simulink model "Simulation_Fahrmodell_v3_straight_line"  (R2023b)
settings: Solver=ode14x  StartTime=0.0  StopTime=600  FixedStep=0.005  RelTol=1e-3
values from neighbouring files (symbols this model uses):
  bat = bat.computePack()    [DoE_main_sensitivity.m]
  cp = cp.computeP4Map(P4, E2, P4_DM, E3, E4)    [DoE_main_sensitivity.m]
  gb = gb.computeShiftMaps()    [DoE_main_sensitivity.m]
  Ice_derfacLoadDecrease_MAP = Ice_derfacLoadDecrease_base    [setup_turbo.m]
  Ice_derfacLoadIncrease_MAP = Ice_derfacLoadIncrease_base    [setup_turbo.m]
  Ice_n_axis = [500, 1000, 1100, 1250, 1320, 1500, 1750, 2000, 2500, 3000, 4500, 6000]    [setup_turbo.m]
  Ice_relLoadMax_CUR_n = [500, 6000]    [setup_turbo.m]
  Ice_relLoadMax_CUR_val = [1.0,  1.0]    [setup_turbo.m]
  Ice_rl_axis_norm = [0.0000, 0.4430, 0.5700, 0.6330, 0.6960, 0.7590, 0.8230, 0.8860, 0.9490, 1.0000]    [setup_turbo.m]
  P4 = cfgNum(cfg, 'P4', 0)    [DoE_main_sensitivity.m]
  P4_DM = cfgNum(cfg, 'P4_DM', 0)    [DoE_main_sensitivity.m]
  pt = pt.setupHybrid()    [DoE_main_sensitivity.m]
  slip_pacejka =     [init_slip.mat]
  use_turbo_model = 0    [setup_turbo.m]
  veh = VehicleConfig()    [DoE_main_sensitivity.m]
undefined symbols (not defined in the file or in its folder): cp_Zelle_JpkgK, seconds, SKO_STREET_CHAL, SKO_WHEEL_TYP_CHAL, T_init_degC, Track, TT_sliced, v_Fzg_init_kmph
libraries: nesl_utility x15, fl_lib x9, simulink x4
(part 4 of 6)

== system Simulation_Fahrmodell_v3_straight_line/Vehicle Dynamics Model /Drivetrain/Primary and Secondary Axle Powertrain Selector/Secondary Axle Powertrain Selector/Auswahl P4, P4_Dual-Motor/No Secondary Axle ==
  n_mot_Upmin : Inport
  Regelfaktor1 : Inport  Port=2
  iAG : Inport  Port=3
  i_ges : Inport  Port=4
  Torque_sh : Inport  Port=5
  Constant : Constant  Value=0
  Terminator{,1..4} (5 alike) : Terminator
  M_Nm GET P4 : Outport
  wires:
  Constant/1 -> M_Nm GET P4/1
  i_ges/1 -> Terminator/1
  iAG/1 -> Terminator1/1
  Regelfaktor1/1 -> Terminator2/1
  n_mot_Upmin/1 -> Terminator3/1
  Torque_sh/1 -> Terminator4/1

== system Simulation_Fahrmodell_v3_straight_line/Vehicle Dynamics Model /Drivetrain/Primary and Secondary Axle Powertrain Selector/Secondary Axle Powertrain Selector/Auswahl P4, P4_Dual-Motor/P4 // E2 Single Motor ==
  n_mot_Upmin : Inport
  Regelfaktor1 : Inport  Port=2
  iAG : Inport  Port=3
  i_ges : Inport  Port=4
  Torque_sh : Inport  Port=5
  1-D Lookup Table1 : Lookup_n-D  NumberOfTableDimensions=1  BreakpointsForDimension1=cp.speed_breakpoints_P4  Table=cp.torque_values_P4  InternalRulePriority=Speed  RndMeth=Simplest
  AG Übersetzung : Product
  Battery and Operating Strategy Limitation (Drive) : Subsystem
  Battery and Operating Strategy Limitation (Recuperation) : Subsystem
  Bus Selector : BusSelector  OutputSignals=tq_sh_P4_des
  Constant : Constant  Value=gb.i_ges_P4
  Constant1 : Constant  Value=gb.i_ges_P4
  Constant5 : Constant  Value=0
  Divide : Product  Inputs=*/
  Gain : Gain  Gain=-1
  Min : MinMax  Inputs=2
  Power Calculation : Subsystem
  "Power Calculation " : Subsystem
  Product : Product
  Relational Operator1 : RelationalOperator  OutDataTypeStr=boolean  RndMeth=Simplest  InputSameDT=off
  Saturation : Saturate  UpperLimit=inf  LowerLimit=0
  Saturation1 : Saturate  UpperLimit=inf  LowerLimit=1
  Smoothing Logic sanfterer Übergang1 : TransferFcn  Denominator=[0.17 1]
  Switch1 : Switch  Criteria=u2 > Threshold  SaturateOnIntegerOverflow=off  InputSameDT=off
  Terminator : Terminator
  M_Nm GET P4 : Outport
  tag scope: P_max_EM_P4_kW=global, P_min_EM_P4_kW=global, tq_sh_P4_max=global
  wires:
  Regelfaktor1/1 -> Relational Operator1/1  "Regelfaktor1"
  Smoothing Logic sanfterer Übergang1/1 -> AG Übersetzung/2
  Relational Operator1/1 -> Switch1/2
  Constant5/1 -> Relational Operator1/2
  Switch1/1 -> Smoothing Logic sanfterer Übergang1/1  "Gesamtmoment motorseitig"
  AG Übersetzung/1 -> M_Nm GET P4/1
  Constant/1 -> AG Übersetzung/1
  iAG/1 -> Terminator/1  "iAG"
  i_ges/1 -> Saturation1/1
  Power Calculation/1(P_kW) -> [P_max_EM_P4_kW]  "P_max_EM_P4_kW"
  Bus Selector/1 -> Saturation/1  "<tq_sh_P4_des>"
  Product/1 -> Battery and Operating Strategy Limitation (Recuperation)/1(Motordrehzahl (1/min)), Battery and Operating Strategy Limitation (Drive)/1(Motordrehzahl (1/min)), 1-D Lookup Table1/1  "Motordrehzahl (1/min)"
  Saturation/1 -> Min/2
  "Power Calculation "/1(P_kW) -> [P_min_EM_P4_kW]  "P_min_EM_P4_kW"
  1-D Lookup Table1/1 -> Gain/1, [tq_sh_P4_max], Min/1
  Torque_sh/1 -> Bus Selector/1
  n_mot_Upmin/1 -> Divide/1  "Motordrehzahl (1/min)"
  Divide/1 -> Product/1  "Motordrehzahl (1/min)"
  Constant1/1 -> Product/2
  Saturation1/1 -> Divide/2
  Battery and Operating Strategy Limitation (Drive)/2(tq_sh_P4_bat_limted) -> Switch1/1, Power Calculation/2(tq_sh_P4_bat_limted)
  Min/1 -> Battery and Operating Strategy Limitation (Drive)/2(Torque_Drive_In)
  [P_max_EM_kW] -> Battery and Operating Strategy Limitation (Drive)/3(P_max_EV_kW)  "P_max_EM_kW"
  Battery and Operating Strategy Limitation (Drive)/1(n_Upmin OUT) -> Power Calculation/1(n_Upmin)
  Battery and Operating Strategy Limitation (Recuperation)/2(tq_sh_P4_bat_limted_recu) -> Switch1/3, "Power Calculation "/2(tq_sh_P4_bat_limted_recu)
  Gain/1 -> Battery and Operating Strategy Limitation (Recuperation)/2(Torque_Recu_In)
  [P_min_EM_kW] -> Battery and Operating Strategy Limitation (Recuperation)/3(P_min_EV_kW)  "P_min_EM_kW"
  Battery and Operating Strategy Limitation (Recuperation)/1(n_Upmin OUT) -> "Power Calculation "/1(n_Upmin)

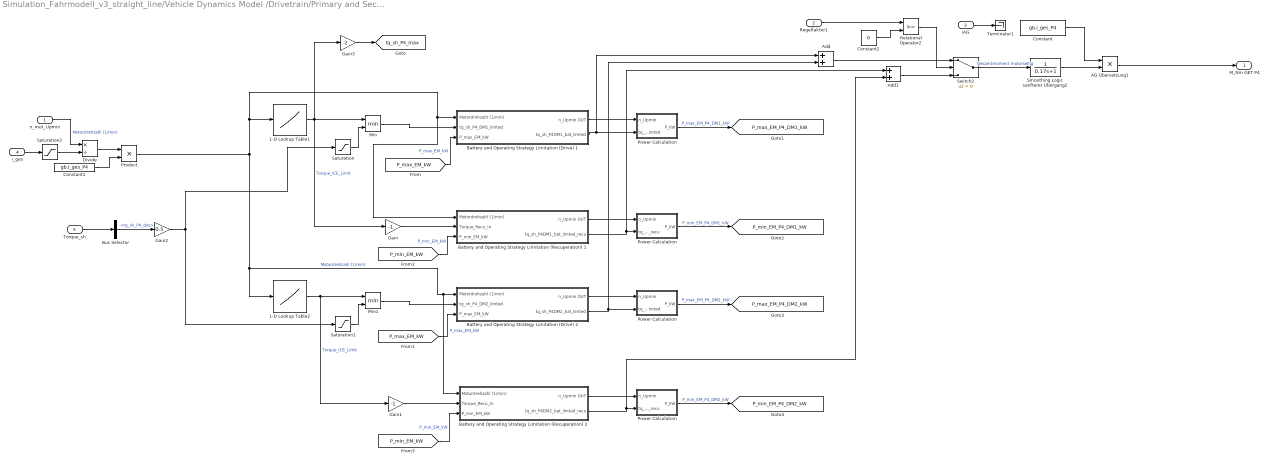
== system Simulation_Fahrmodell_v3_straight_line/Vehicle Dynamics Model /Drivetrain/Primary and Secondary Axle Powertrain Selector/Secondary Axle Powertrain Selector/Auswahl P4, P4_Dual-Motor/P4 // E3 // E4 Dual Motor ==
  n_mot_Upmin : Inport
  Regelfaktor1 : Inport  Port=2
  iAG : Inport  Port=3
  i_ges : Inport  Port=4
  Torque_sh : Inport  Port=5
  1-D Lookup Table1 : Lookup_n-D  NumberOfTableDimensions=1  BreakpointsForDimension1=cp.speed_breakpoints_P4  Table=cp.torque_values_P4  InternalRulePriority=Speed  RndMeth=Simplest
  1-D Lookup Table2 : Lookup_n-D  NumberOfTableDimensions=1  BreakpointsForDimension1=cp.speed_breakpoints_P4  Table=cp.torque_values_P4  InternalRulePriority=Speed  RndMeth=Simplest
  AG Übersetzung1 : Product
  Add : Sum
  Add1 : Sum
  Battery and Operating Strategy Limitation (Drive) 1 : Subsystem
  Battery and Operating Strategy Limitation (Drive) 2 : Subsystem
  Battery and Operating Strategy Limitation (Recuperation) 1 : Subsystem
  Battery and Operating Strategy Limitation (Recuperation) 2 : Subsystem
  Bus Selector : BusSelector  OutputSignals=tq_sh_P4_des
  Constant : Constant  Value=gb.i_ges_P4
  Constant1 : Constant  Value=gb.i_ges_P4
  Constant2 : Constant  Value=0
  Divide : Product  Inputs=*/
  Gain : Gain  Gain=-1
  Gain1 : Gain  Gain=-1
  Gain2 : Gain  Gain=0.5
  Gain3 : Gain  Gain=2
  Min : MinMax  Inputs=2
  Min1 : MinMax  Inputs=2
  "Power Calculation " : Subsystem
  "Power Calculation   " : Subsystem
  "Power Calculation    " : Subsystem
  "Power Calculation     " : Subsystem
  Product : Product
  Relational Operator2 : RelationalOperator  OutDataTypeStr=boolean  RndMeth=Simplest  InputSameDT=off
  Saturation : Saturate  UpperLimit=inf  LowerLimit=0
  Saturation1 : Saturate  UpperLimit=inf  LowerLimit=0
  Saturation2 : Saturate  UpperLimit=inf  LowerLimit=1
  Smoothing Logic sanfterer Übergang2 : TransferFcn  Denominator=[0.17 1]
  Switch2 : Switch  Criteria=u2 > Threshold  SaturateOnIntegerOverflow=off  InputSameDT=off
  Terminator1 : Terminator
  M_Nm GET P4 : Outport
  tag scope: P_max_EM_P4_DM1_kW=global, P_max_EM_P4_DM2_kW=global, P_min_EM_P4_DM1_kW=global, P_min_EM_P4_DM2_kW=global, tq_sh_P4_max=global
  wires:
  Bus Selector/1 -> Gain2/1  "<tq_sh_P4_des>"
  "Power Calculation    "/1(P_kW) -> [P_min_EM_P4_DM1_kW]  "P_min_EM_P4_DM1_kW"
  Torque_sh/1 -> Bus Selector/1
  "Power Calculation     "/1(P_kW) -> [P_max_EM_P4_DM1_kW]  "P_max_EM_P4_DM1_kW"
  1-D Lookup Table1/1 -> Gain3/1, Min/1, Gain/1  "Torque_ICE_Limit"
  Saturation/1 -> Min/2
  "Power Calculation "/1(P_kW) -> [P_min_EM_P4_DM2_kW]  "P_min_EM_P4_DM2_kW"
  "Power Calculation   "/1(P_kW) -> [P_max_EM_P4_DM2_kW]  "P_max_EM_P4_DM2_kW"
  1-D Lookup Table2/1 -> Gain1/1, Min1/1  "Torque_ICE_Limit"
  Saturation1/1 -> Min1/2
  AG Übersetzung1/1 -> M_Nm GET P4/1
  Constant/1 -> AG Übersetzung1/1
  Switch2/1 -> Smoothing Logic sanfterer Übergang2/1  "Gesamtmoment motorseitig"
  iAG/1 -> Terminator1/1
  Relational Operator2/1 -> Switch2/2
  Regelfaktor1/1 -> Relational Operator2/1
  Add1/1 -> Switch2/3
  Constant2/1 -> Relational Operator2/2
  Add/1 -> Switch2/1
  Smoothing Logic sanfterer Übergang2/1 -> AG Übersetzung1/2
  Gain2/1 -> Saturation/1, Saturation1/1
  n_mot_Upmin/1 -> Divide/1  "Motordrehzahl (1/min)"
  i_ges/1 -> Saturation2/1
  Divide/1 -> Product/1
  Constant1/1 -> Product/2
  Product/1 -> Battery and Operating Strategy Limitation (Recuperation) 1/1(Motordrehzahl (1/min)), Battery and Operating Strategy Limitation (Drive) 1/1(Motordrehzahl (1/min)), 1-D Lookup Table1/1, 1-D Lookup Table2/1, Battery and Operating Strategy Limitation (Recuperation) 2/1(Motordrehzahl (1/min)), Battery and Operating Strategy Limitation (Drive) 2/1(Motordrehzahl (1/min))  "Motordrehzahl (1/min)"
  Saturation2/1 -> Divide/2
  Gain3/1 -> [tq_sh_P4_max]
  Battery and Operating Strategy Limitation (Drive) 1/2(tq_sh_P4DM1_bat_limted) -> Add/1, "Power Calculation     "/2(tq_sh_P4DM1_bat_limted)
  Min/1 -> Battery and Operating Strategy Limitation (Drive) 1/2(tq_sh_P4_DM1_limted)
  [P_max_EM_kW] -> Battery and Operating Strategy Limitation (Drive) 1/3(P_max_EM_kW)  "P_max_EM_kW"
  Battery and Operating Strategy Limitation (Drive) 1/1(n_Upmin OUT) -> "Power Calculation     "/1(n_Upmin)
  Battery and Operating Strategy Limitation (Recuperation) 1/2(tq_sh_P4DM1_bat_limted_recu) -> Add1/1, "Power Calculation    "/2(tq_sh_P4DM1_bat_limted_recu)
  Gain/1 -> Battery and Operating Strategy Limitation (Recuperation) 1/2(Torque_Recu_In)
  [P_min_EM_kW] -> Battery and Operating Strategy Limitation (Recuperation) 1/3(P_min_EM_kW)  "P_min_EM_kW"
  Battery and Operating Strategy Limitation (Recuperation) 1/1(n_Upmin OUT) -> "Power Calculation    "/1(n_Upmin)
  Battery and Operating Strategy Limitation (Drive) 2/2(tq_sh_P4DM2_bat_limted) -> Add/2, "Power Calculation   "/2(tq_sh_P4DM2_bat_limted)
  Min1/1 -> Battery and Operating Strategy Limitation (Drive) 2/2(tq_sh_P4_DM2_limted)
  [P_max_EM_kW] -> Battery and Operating Strategy Limitation (Drive) 2/3(P_max_EM_kW)  "P_max_EM_kW"
  Battery and Operating Strategy Limitation (Drive) 2/1(n_Upmin OUT) -> "Power Calculation   "/1(n_Upmin)
  Battery and Operating Strategy Limitation (Recuperation) 2/2(tq_sh_P4DM2_bat_limted_recu) -> Add1/2, "Power Calculation "/2(tq_sh_P4DM2_bat_limted_recu)
  Gain1/1 -> Battery and Operating Strategy Limitation (Recuperation) 2/2(Torque_Recu_In)
  [P_min_EM_kW] -> Battery and Operating Strategy Limitation (Recuperation) 2/3(P_min_EM_kW)  "P_min_EM_kW"
  Battery and Operating Strategy Limitation (Recuperation) 2/1(n_Upmin OUT) -> "Power Calculation "/1(n_Upmin)

== system Simulation_Fahrmodell_v3_straight_line/Vehicle Dynamics Model /Drivetrain/GETRIEBE auswahl VK, EV/Transmission Selector/ICE Multi-Speed/Simulation Doppelkupplung (Gangwechsel ohne Zugkraftunterbrechung) orig2/Vorheriger Wert ==
  In1 : Inport
  Delay : Delay  DelayLength=1
  Memory : Memory
  Relational Operator : RelationalOperator  Operator=~=  OutDataTypeStr=boolean  RndMeth=Simplest  InputSameDT=off
  Switch1 : Switch  Criteria=u2 > Threshold  SaturateOnIntegerOverflow=off  InputSameDT=off
  Out1 : Outport
  wires:
  Switch1/1 -> Memory/1, Out1/1
  Relational Operator/1 -> Switch1/2
  Delay/1 -> Relational Operator/2, Switch1/1
  In1/1 -> Relational Operator/1, Delay/1
  Memory/1 -> Switch1/3

== system Simulation_Fahrmodell_v3_straight_line/Vehicle Dynamics Model /Drivetrain/GETRIEBE auswahl VK, EV/Transmission Selector/ICE Multi-Speed/Subsystem1/Desired Gear  ==
  Current Gear : Inport
  Upshift_Signal : Inport  Port=2
  cmd : Inport  Port=3
  Downshift_Signal : Inport  Port=4
  Add : Sum
  Add1 : Sum  Inputs=+-
  Begrenzung Gang : Saturate  UpperLimit=gb.No_Gears  LowerLimit=1
  Constant1 : Constant
  Constant2 : Constant
  Constant6 : Constant  Value=0
  Relational Operator1 : RelationalOperator  Operator===  OutDataTypeStr=boolean  RndMeth=Simplest  InputSameDT=off
  Switch{1,3..5} (4 alike) : Switch  Criteria=u2 > Threshold  SaturateOnIntegerOverflow=off  InputSameDT=off
  Unit Delay : UnitDelay  SampleTime=0.005
  desiredGear : Outport
  wires:
  Add1/1 -> Switch4/1
  Current Gear/1 -> Add1/1, Switch4/3, Switch3/3, Add/1, Switch1/1
  Switch1/1 -> Begrenzung Gang/1  "Current_Gear"
  Constant1/1 -> Add/2
  Add/1 -> Switch3/1
  Upshift_Signal/1 -> Switch3/2
  Switch4/1 -> Switch5/3
  cmd/1 -> Switch5/2, Relational Operator1/1
  Switch3/1 -> Switch5/1
  Relational Operator1/1 -> Switch1/2
  Unit Delay/1 -> desiredGear/1
  Switch5/1 -> Switch1/3  "Current_Gear"
  Constant6/1 -> Relational Operator1/2
  Constant2/1 -> Add1/2
  Begrenzung Gang/1 -> Unit Delay/1  "Normal"
  Downshift_Signal/1 -> Switch4/2

== system Simulation_Fahrmodell_v3_straight_line/Vehicle Dynamics Model /Drivetrain/GETRIEBE auswahl VK, EV/Transmission Selector/ICE Multi-Speed/Subsystem1/Locktime Bypass Conditions  ==
  note: FOR DOWNSHIFT
  note: FOR UPSHIFT
  Gear upshift Rpm : Inport
  Current Rpm : Inport  Port=2
  Gear downshift Rpm : Inport  Port=3
  AND : Logic  IconShape=distinctive  AllPortsSameDT=off  OutDataTypeStr=boolean
  AND1 : Logic  IconShape=distinctive  AllPortsSameDT=off  OutDataTypeStr=boolean
  AND2 : Logic  IconShape=distinctive  AllPortsSameDT=off  OutDataTypeStr=boolean
  Constant{4..5,7..8} (4 alike) : Constant  Value=0
  OR : Logic  Operator=OR  IconShape=distinctive  AllPortsSameDT=off  OutDataTypeStr=boolean
  OR1 : Logic  Operator=OR  IconShape=distinctive  AllPortsSameDT=off  OutDataTypeStr=boolean
  Relational Operator2 : RelationalOperator  Operator=>  OutDataTypeStr=boolean  RndMeth=Simplest  InputSameDT=off
  Relational Operator5 : RelationalOperator  Operator=<=  OutDataTypeStr=boolean  RndMeth=Simplest  InputSameDT=off
  Relational Operator6 : RelationalOperator  Operator=<=  OutDataTypeStr=boolean  RndMeth=Simplest  InputSameDT=off
  Relational Operator7 : RelationalOperator  OutDataTypeStr=boolean  RndMeth=Simplest  InputSameDT=off
  Relational Operator8 : RelationalOperator  Operator=>  OutDataTypeStr=boolean  RndMeth=Simplest  InputSameDT=off
  Relational Operator9 : RelationalOperator  Operator=<=  OutDataTypeStr=boolean  RndMeth=Simplest  InputSameDT=off
  cmd_Bypass_Lock_time : Outport
  wires:
  Constant8/1 -> Relational Operator9/2
  Relational Operator5/1 -> AND1/1
  [Gaspedalposition] -> Relational Operator5/1, Relational Operator8/1, Relational Operator2/1  "Gas Pedal Position"
  Relational Operator7/1 -> AND/2
  Relational Operator2/1 -> AND/1
  Relational Operator6/1 -> AND1/2
  Gear downshift Rpm/1 -> Relational Operator6/2
  Constant4/1 -> Relational Operator2/2
  Current Rpm/1 -> Relational Operator7/1, Relational Operator6/1
  AND1/1 -> OR/1
  Constant7/1 -> Relational Operator8/2
  OR/1 -> OR1/2  "Bypass Lock time"
  AND/1 -> OR1/1  "Bypass Lock time"
  Constant5/1 -> Relational Operator5/2
  AND2/1 -> OR/2
  Relational Operator8/1 -> AND2/1
  Relational Operator9/1 -> AND2/2
  [S_BUS_IST_Profil_a] -> Relational Operator9/1  "Acceleration"
  OR1/1 -> cmd_Bypass_Lock_time/1  "cmd_Bypass_Lock_time"
  Gear upshift Rpm/1 -> Relational Operator7/2

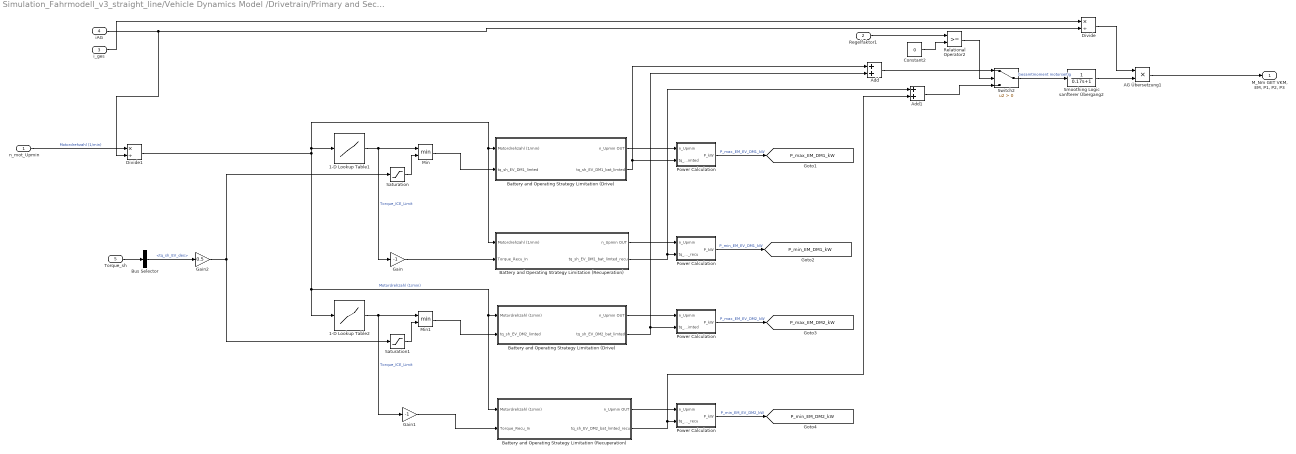
== system Simulation_Fahrmodell_v3_straight_line/Vehicle Dynamics Model /Drivetrain/Primary and Secondary Axle Powertrain Selector/Primary Axle Powertrain Selector/Electric Drive/Variant Subsystem/EV Dual Motor ==
  n_mot_Upmin : Inport
  Regelfaktor1 : Inport  Port=2
  i_ges : Inport  Port=3
  iAG : Inport  Port=4
  Torque_sh : Inport  Port=5
  1-D Lookup Table1 : Lookup_n-D  NumberOfTableDimensions=1  BreakpointsForDimension1=cp.speed_breakpoints_EV  Table=cp.torque_values_EV  InternalRulePriority=Speed  RndMeth=Simplest
  1-D Lookup Table2 : Lookup_n-D  NumberOfTableDimensions=1  BreakpointsForDimension1=cp.speed_breakpoints_EV  Table=cp.torque_values_EV  InternalRulePriority=Speed  RndMeth=Simplest
  AG Übersetzung1 : Product
  Add : Sum
  Add1 : Sum
  Battery and Operating Strategy Limitation (Drive) : Subsystem
  "Battery and Operating Strategy Limitation (Drive) " : Subsystem
  Battery and Operating Strategy Limitation (Recuperation) : Subsystem
  "Battery and Operating Strategy Limitation (Recuperation) " : Subsystem
  Bus Selector : BusSelector  OutputSignals=tq_sh_EV_des
  Constant2 : Constant  Value=0
  Divide : Product  Inputs=*/
  Divide1 : Product  Inputs=*/
  Gain : Gain  Gain=-1
  Gain1 : Gain  Gain=-1
  Gain2 : Gain  Gain=0.5
  Min : MinMax  Inputs=2
  Min1 : MinMax  Inputs=2
  Power Calculation : Subsystem
  "Power Calculation " : Subsystem
  "Power Calculation  " : Subsystem
  "Power Calculation    " : Subsystem
  Relational Operator2 : RelationalOperator  OutDataTypeStr=boolean  RndMeth=Simplest  InputSameDT=off
  Saturation : Saturate  UpperLimit=inf  LowerLimit=0
  Saturation1 : Saturate  UpperLimit=inf  LowerLimit=0
  Smoothing Logic sanfterer Übergang2 : TransferFcn  Denominator=[0.17 1]
  Switch2 : Switch  Criteria=u2 > Threshold  SaturateOnIntegerOverflow=off  InputSameDT=off
  "M_Nm GET VKM, EM, P1, P2, P3" : Outport
  tag scope: P_max_EM_DM1_kW=global, P_max_EM_DM2_kW=global, P_min_EM_DM1_kW=global, P_min_EM_DM2_kW=global
  wires:
  Add1/1 -> Switch2/3
  Add/1 -> Switch2/1
  Switch2/1 -> Smoothing Logic sanfterer Übergang2/1  "Gesamtmoment motorseitig"
  Smoothing Logic sanfterer Übergang2/1 -> AG Übersetzung1/2
  Regelfaktor1/1 -> Relational Operator2/1
  Relational Operator2/1 -> Switch2/2
  AG Übersetzung1/1 -> "M_Nm GET VKM, EM, P1, P2, P3"/1
  Constant2/1 -> Relational Operator2/2
  i_ges/1 -> Divide/1
  iAG/1 -> Divide1/2, Divide/2
  Divide/1 -> AG Übersetzung1/1
  Saturation1/1 -> Min1/2
  "Power Calculation    "/1(P_kW) -> [P_max_EM_DM2_kW]  "P_max_EM_EV_DM2_kW"
  1-D Lookup Table2/1 -> Gain1/1, Min1/1  "Torque_ICE_Limit"
  "Power Calculation  "/1(P_kW) -> [P_min_EM_DM1_kW]  "P_min_EM_EV_DM1_kW"
  "Power Calculation "/1(P_kW) -> [P_max_EM_DM1_kW]  "P_max_EM_EV_DM1_kW"
  Divide1/1 -> 1-D Lookup Table2/1, "Battery and Operating Strategy Limitation (Recuperation) "/1(Motordrehzahl (1/min)), "Battery and Operating Strategy Limitation (Drive) "/1(Motordrehzahl (1/min)), Battery and Operating Strategy Limitation (Recuperation)/1(Motordrehzahl (1/min)), Battery and Operating Strategy Limitation (Drive)/1(Motordrehzahl (1/min)), 1-D Lookup Table1/1  "Motordrehzahl (1/min)"
  Power Calculation/1(P_kW) -> [P_min_EM_DM2_kW]  "P_min_EM_EV_DM2_kW"
  Gain2/1 -> Saturation1/1, Saturation/1
  Saturation/1 -> Min/2
  1-D Lookup Table1/1 -> Gain/1, Min/1  "Torque_ICE_Limit"
  Torque_sh/1 -> Bus Selector/1
  Bus Selector/1 -> Gain2/1  "<tq_sh_EV_des>"
  n_mot_Upmin/1 -> Divide1/1  "Motordrehzahl (1/min)"
  Battery and Operating Strategy Limitation (Drive)/2(tq_sh_EV_DM1_bat_limted) -> Add/1, "Power Calculation "/2(tq_sh_EV_DM1_bat_limted)
  Min/1 -> Battery and Operating Strategy Limitation (Drive)/2(tq_sh_EV_DM1_limted)
  Battery and Operating Strategy Limitation (Drive)/1(n_Upmin OUT) -> "Power Calculation "/1(n_Upmin)
  Battery and Operating Strategy Limitation (Recuperation)/2(tq_sh_EV_DM1_bat_limted_recu) -> Add1/1, "Power Calculation  "/2(tq_sh_EV_DM1_bat_limted_recu)
  Gain/1 -> Battery and Operating Strategy Limitation (Recuperation)/2(Torque_Recu_In)
  Battery and Operating Strategy Limitation (Recuperation)/1(n_Upmin OUT) -> "Power Calculation  "/1(n_Upmin)
  "Battery and Operating Strategy Limitation (Drive) "/2(tq_sh_EV_DM2_bat_limted) -> Add/2, "Power Calculation    "/2(tq_sh_EV_DM2_bat_limted)
  Min1/1 -> "Battery and Operating Strategy Limitation (Drive) "/2(tq_sh_EV_DM2_limted)
  "Battery and Operating Strategy Limitation (Drive) "/1(n_Upmin OUT) -> "Power Calculation    "/1(n_Upmin)
  "Battery and Operating Strategy Limitation (Recuperation) "/2(tq_sh_EV_DM2_bat_limted_recu) -> Add1/2, Power Calculation/2(tq_sh_EV_DM2_bat_limted_recu)
  Gain1/1 -> "Battery and Operating Strategy Limitation (Recuperation) "/2(Torque_Recu_In)
  "Battery and Operating Strategy Limitation (Recuperation) "/1(n_Upmin OUT) -> Power Calculation/1(n_Upmin)

== system Simulation_Fahrmodell_v3_straight_line/Vehicle Dynamics Model /Drivetrain/Primary and Secondary Axle Powertrain Selector/Primary Axle Powertrain Selector/Electric Drive/Variant Subsystem/EV Single Motor ==
  Regelfaktor1 : Inport
  n_mot_Upmin : Inport  Port=2
  i_ges : Inport  Port=3
  iAG : Inport  Port=4
  Torque_sh : Inport  Port=5
  1-D Lookup Table1 : Lookup_n-D  NumberOfTableDimensions=1  BreakpointsForDimension1=cp.speed_breakpoints_EV  Table=cp.torque_values_EV  InternalRulePriority=Speed  RndMeth=Simplest
  Battery and Operating Strategy Limitation (Drive) : Subsystem
  Battery and Operating Strategy Limitation (Recuperation) : Subsystem
  Bus Selector : BusSelector  OutputSignals=tq_sh_EV_des
  Constant7 : Constant  Value=0
  Gain : Gain  Gain=-1
  Min : MinMax  Inputs=2
  Power Calculation : Subsystem
  "Power Calculation " : Subsystem
  Relational Operator2 : RelationalOperator  OutDataTypeStr=boolean  RndMeth=Simplest  InputSameDT=off
  Saturation : Saturate  UpperLimit=inf  LowerLimit=0
  Smoothing Logic sanfterer Übergang2 : TransferFcn  Denominator=[0.17 1]
  Switch2 : Switch  Criteria=u2 > Threshold  SaturateOnIntegerOverflow=off  InputSameDT=off
  Terminator : Terminator
  Wirkungsgrad Antriebsstrang1 : Subsystem
  i_GES Übersetzung : Product
  "M_Nm GET VKM, EM, P1, P2, P3" : Outport
  tag scope: P_max_EM_EV_kW=global, P_min_EM_EV_kW=global
  wires:
  iAG/1 -> Terminator/1
  Constant7/1 -> Relational Operator2/2
  Smoothing Logic sanfterer Übergang2/1 -> i_GES Übersetzung/2
  Switch2/1 -> Smoothing Logic sanfterer Übergang2/1  "Gesamtmoment motorseitig"
  Wirkungsgrad Antriebsstrang1/1(M_Nm OUT) -> "M_Nm GET VKM, EM, P1, P2, P3"/1
  Relational Operator2/1 -> Switch2/2
  Regelfaktor1/1 -> Relational Operator2/1
  i_GES Übersetzung/1 -> Wirkungsgrad Antriebsstrang1/1(M_Nm IN)
  i_ges/1 -> i_GES Übersetzung/1  "i_GES"
  n_mot_Upmin/1 -> Battery and Operating Strategy Limitation (Recuperation)/1(Motordrehzahl (1/min)), Battery and Operating Strategy Limitation (Drive)/1(Motordrehzahl (1/min)), 1-D Lookup Table1/1  "Motordrehzahl (1/min)"
  Power Calculation/1(P_kW) -> [P_max_EM_EV_kW]  "P_max_EM_EV_kW"
  1-D Lookup Table1/1 -> Min/1, Gain/1  "Torque_ICE_Limit"
  Saturation/1 -> Min/2
  Bus Selector/1 -> Saturation/1  "<tq_sh_EV_des>"
  "Power Calculation "/1(P_kW) -> [P_min_EM_EV_kW]  "P_min_EM_EV_kW"
  Torque_sh/1 -> Bus Selector/1
  Battery and Operating Strategy Limitation (Drive)/2(tq_sh_EM_bat_limted) -> Switch2/1, Power Calculation/2(tq_sh_EM_bat_limted)
  Min/1 -> Battery and Operating Strategy Limitation (Drive)/2(tq_sh_EM_limted)  "tq_sh_EM_limted"
  Battery and Operating Strategy Limitation (Drive)/1(n_Upmin OUT) -> Power Calculation/1(n_Upmin)
  Battery and Operating Strategy Limitation (Recuperation)/2(tq_sh_EM_bat_limted_recu) -> Switch2/3, "Power Calculation "/2(tq_sh_EM_bat_limted_recu)
  Gain/1 -> Battery and Operating Strategy Limitation (Recuperation)/2(Torque_Recu_In)
  Battery and Operating Strategy Limitation (Recuperation)/1(n_Upmin OUT) -> "Power Calculation "/1(n_Upmin)

== system Simulation_Fahrmodell_v3_straight_line/Vehicle Dynamics Model /Drivetrain/Primary and Secondary Axle Powertrain Selector/Primary Axle Powertrain Selector/Hybrid Drive/ICE/Berechnung Leistung 1 ==
  n_Upmin : Inport
  M_Nm : Inport  Port=2
  Constant1 : Constant  Value=2*pi/60/1000
  Product : Product  Inputs=3
  P_kW : Outport
  wires:
  Product/1 -> P_kW/1
  n_Upmin/1 -> Product/2
  Constant1/1 -> Product/3
  M_Nm/1 -> Product/1

== system Simulation_Fahrmodell_v3_straight_line/Vehicle Dynamics Model /Drivetrain/Primary and Secondary Axle Powertrain Selector/Primary Axle Powertrain Selector/Hybrid Drive/ICE/Berechnung Leistung 4 ==
  n_Upmin : Inport
  M_Nm : Inport  Port=2
  Constant1 : Constant  Value=2*pi/60/1000
  Product : Product  Inputs=3
  P_kW : Outport
  wires:
  Product/1 -> P_kW/1
  n_Upmin/1 -> Product/2
  Constant1/1 -> Product/3
  M_Nm/1 -> Product/1

== system Simulation_Fahrmodell_v3_straight_line/Vehicle Dynamics Model /Drivetrain/Primary and Secondary Axle Powertrain Selector/Primary Axle Powertrain Selector/Hybrid Drive/ICE/Turbo Lag (Beta) ==
  Torque_ICE_Limit : Inport
  Motordrehzahl (1/min) : Inport  Port=2
  Constant1 : Constant  Value=use_turbo_model
  Product : Product
  Switch : Switch  Criteria=u2 > Threshold  SaturateOnIntegerOverflow=off  InputSameDT=off
  Turbo Lag : Subsystem
  Out1 : Outport
  wires:
  Motordrehzahl (1/min)/1 -> Turbo Lag/1(n_ICE)
  Switch/1 -> Out1/1
  Product/1 -> Switch/1
  Torque_ICE_Limit/1 -> Product/2, Switch/3
  Constant1/1 -> Switch/2
  Turbo Lag/1(rl) -> Product/1
  [Gaspedalposition] -> Turbo Lag/2(rl_des)

== system Simulation_Fahrmodell_v3_straight_line/Vehicle Dynamics Model /Drivetrain/Primary and Secondary Axle Powertrain Selector/Primary Axle Powertrain Selector/Hybrid Drive/P0/P0 Motor ==
  n_Upmin IN : Inport
  Torque_P0_sh : Inport  Port=2
  P_max_EM_kW : Inport  Port=3
  P_min_EM_kW : Inport  Port=4
  1-D Lookup Table1 : Lookup_n-D  NumberOfTableDimensions=1  BreakpointsForDimension1=cp.speed_breakpoints_P0  Table=cp.torque_values_P0  InternalRulePriority=Speed  RndMeth=Simplest
  Battery and Operating Strategy Limitation (Recuperation) : Subsystem
  Gain : Gain  Gain=-1
  Min : MinMax  Inputs=2
  Power Calculation : Subsystem
  "Power Calculation " : Subsystem
  Saturation : Saturate  UpperLimit=inf  LowerLimit=0
  SubsysteBattery and Operating Strategy Limitation (Drive)m : Subsystem
  P0_M_Nm_Fahren : Outport
  P_max_EM_P0_kW : Outport  Port=2
  P_min_EM_P0_kW : Outport  Port=3
  P0_M_Nm_Reku : Outport  Port=4
  tag scope: tq_sh_P0_max=global
  wires:
  Power Calculation/1(P_kW) -> P_max_EM_P0_kW/1
  "Power Calculation "/1(P_kW) -> P_min_EM_P0_kW/1
  Saturation/1 -> Min/2
  1-D Lookup Table1/1 -> Gain/1, [tq_sh_P0_max], Min/1  "Torque_ICE_Limit"
  n_Upmin IN/1 -> Battery and Operating Strategy Limitation (Recuperation)/1(Motordrehzahl (1/min)), SubsysteBattery and Operating Strategy Limitation (Drive)m/1(Motordrehzahl (1/min)), 1-D Lookup Table1/1  "Motordrehzahl (1/min)"
  Torque_P0_sh/1 -> Saturation/1
  SubsysteBattery and Operating Strategy Limitation (Drive)m/2(tq_sh_P0_bat_limted) -> P0_M_Nm_Fahren/1, Power Calculation/2(tq_sh_P0_bat_limted)
  Min/1 -> SubsysteBattery and Operating Strategy Limitation (Drive)m/2(tq_sh_P0_limted)  "tq_sh_P0_limted"
  P_max_EM_kW/1 -> SubsysteBattery and Operating Strategy Limitation (Drive)m/3(P_mech_max_kW)
  SubsysteBattery and Operating Strategy Limitation (Drive)m/1(n_Upmin OUT) -> Power Calculation/1(n_Upmin)
  Battery and Operating Strategy Limitation (Recuperation)/2(tq_sh_P0_bat_limted_recu) -> P0_M_Nm_Reku/1, "Power Calculation "/2(tq_sh_P0_bat_limted_recu)
  Gain/1 -> Battery and Operating Strategy Limitation (Recuperation)/2(Torque_Recu_In)
  P_min_EM_kW/1 -> Battery and Operating Strategy Limitation (Recuperation)/3(P_mech_max_kW)
  Battery and Operating Strategy Limitation (Recuperation)/1(n_Upmin OUT) -> "Power Calculation "/1(n_Upmin)

== system Simulation_Fahrmodell_v3_straight_line/Vehicle Dynamics Model /Drivetrain/Primary and Secondary Axle Powertrain Selector/Primary Axle Powertrain Selector/Hybrid Drive/P0/P0 Motor disabled ==
  n_Upmin IN : Inport
  Torque_P0_sh : Inport  Port=2
  P_max_EM_kW : Inport  Port=3
  P_min_EM_kW : Inport  Port=4
  Constant : Constant  Value=0
  Terminator{,1..3} (4 alike) : Terminator
  P0_M_Nm_Fahren : Outport
  P_max_EM_P0_kW : Outport  Port=2
  P_min_EM_P0_kW : Outport  Port=3
  P0_M_Nm_Reku : Outport  Port=4
  wires:
  Constant/1 -> P_min_EM_P0_kW/1, P_max_EM_P0_kW/1, P0_M_Nm_Fahren/1, P0_M_Nm_Reku/1
  n_Upmin IN/1 -> Terminator/1  "Motordrehzahl (1/min)"
  P_max_EM_kW/1 -> Terminator1/1
  P_min_EM_kW/1 -> Terminator2/1
  Torque_P0_sh/1 -> Terminator3/1

== system Simulation_Fahrmodell_v3_straight_line/Vehicle Dynamics Model /Drivetrain/Primary and Secondary Axle Powertrain Selector/Primary Axle Powertrain Selector/Hybrid Drive/P2/P2 Motor ==
  n_Upmin IN : Inport
  Torque_P2_sh : Inport  Port=2
  P_max_EM_kW : Inport  Port=3
  P_min_EM_kW : Inport  Port=4
  1-D Lookup Table1 : Lookup_n-D  NumberOfTableDimensions=1  BreakpointsForDimension1=cp.speed_breakpoints_P2  Table=cp.torque_values_P2  InternalRulePriority=Speed  RndMeth=Simplest
  Battery and Operating Strategy Limitation (Drive) : Subsystem
  Battery and Operating Strategy Limitation (Recuperation) : Subsystem
  Gain : Gain  Gain=-1
  Min : MinMax  Inputs=2
  Power Calculation : Subsystem
  "Power Calculation " : Subsystem
  Saturation : Saturate  UpperLimit=inf  LowerLimit=0
  P2_M_Nm_Fahren : Outport
  P_max_EM_P2_kW : Outport  Port=2
  P_min_EM_P2_kW : Outport  Port=3
  P2_M_Nm_Reku : Outport  Port=4
  tag scope: tq_sh_P2_max=global
  wires:
  Power Calculation/1(P_kW) -> P_max_EM_P2_kW/1  "P_max_EM_P2_kW"
  "Power Calculation "/1(P_kW) -> P_min_EM_P2_kW/1  "P_min_EM_P2_kW"
  Saturation/1 -> Min/2
  1-D Lookup Table1/1 -> Min/1, [tq_sh_P2_max], Gain/1  "Torque_ICE_Limit"
  n_Upmin IN/1 -> Battery and Operating Strategy Limitation (Recuperation)/1(Motordrehzahl (1/min)), Battery and Operating Strategy Limitation (Drive)/1(Motordrehzahl (1/min)), 1-D Lookup Table1/1  "Motordrehzahl (1/min)"
  Torque_P2_sh/1 -> Saturation/1
  Battery and Operating Strategy Limitation (Drive)/2(tq_sh_P2_bat_limted) -> P2_M_Nm_Fahren/1, Power Calculation/2(tq_sh_P2_bat_limted)
  Min/1 -> Battery and Operating Strategy Limitation (Drive)/2(tq_sh_P2_limted)  "tq_sh_P2_limted"
  P_max_EM_kW/1 -> Battery and Operating Strategy Limitation (Drive)/3(P_max_EM_kW)  "P_max_EM_kW"
  Battery and Operating Strategy Limitation (Drive)/1(n_Upmin OUT) -> Power Calculation/1(n_Upmin)
  Battery and Operating Strategy Limitation (Recuperation)/2(tq_sh_P2_bat_limted_recu) -> P2_M_Nm_Reku/1, "Power Calculation "/2(tq_sh_P2_bat_limted_recu)
  Gain/1 -> Battery and Operating Strategy Limitation (Recuperation)/2(Torque_Recu_In)
  P_min_EM_kW/1 -> Battery and Operating Strategy Limitation (Recuperation)/3(P_min_EM_kW)  "P_min_EM_kW"
  Battery and Operating Strategy Limitation (Recuperation)/1(n_Upmin OUT) -> "Power Calculation "/1(n_Upmin)

== system Simulation_Fahrmodell_v3_straight_line/Vehicle Dynamics Model /Drivetrain/Primary and Secondary Axle Powertrain Selector/Primary Axle Powertrain Selector/Hybrid Drive/P2/P2 Motor disabled ==
  n_Upmin IN : Inport
  Torque_P2_sh : Inport  Port=2
  P_max_EM_kW : Inport  Port=3
  P_min_EM_kW : Inport  Port=4
  Constant : Constant  Value=0
  Terminator{,1..3} (4 alike) : Terminator
  P2_M_Nm_Fahren : Outport
  P_max_EM_P2_kW : Outport  Port=2
  P_min_EM_P2_kW : Outport  Port=3
  P2_M_Nm_Reku : Outport  Port=4
  wires:
  Constant/1 -> P_min_EM_P2_kW/1, P_max_EM_P2_kW/1, P2_M_Nm_Fahren/1, P2_M_Nm_Reku/1
  n_Upmin IN/1 -> Terminator/1  "Motordrehzahl (1/min)"
  P_max_EM_kW/1 -> Terminator1/1
  P_min_EM_kW/1 -> Terminator2/1
  Torque_P2_sh/1 -> Terminator3/1

== system Simulation_Fahrmodell_v3_straight_line/Vehicle Dynamics Model /Drivetrain/Primary and Secondary Axle Powertrain Selector/Primary Axle Powertrain Selector/Hybrid Drive/P3/P3 Motor ==
  n_Upmin IN : Inport
  tq_sh_P3_des : Inport  Port=2
  P_max_EM_kW : Inport  Port=3
  P_min_EM_kW : Inport  Port=4
  1-D Lookup Table1 : Lookup_n-D  NumberOfTableDimensions=1  BreakpointsForDimension1=cp.speed_breakpoints_P3  Table=cp.torque_values_P3  InternalRulePriority=Speed  RndMeth=Simplest
  Battery and Operating Strategy Limitation (Drive) : Subsystem
  Battery and Operating Strategy Limitation (Recuperation) : Subsystem
  Gain : Gain  Gain=-1
  Min : MinMax  Inputs=2
  Power Calculation : Subsystem
  "Power Calculation " : Subsystem
  Saturation : Saturate  UpperLimit=inf  LowerLimit=0
  P3_M_Nm_Drive : Outport
  P_max_EM_P3_kW : Outport  Port=2
  P_min_EM_P3_kW : Outport  Port=3
  P3_M_Nm_Recu : Outport  Port=4
  tag scope: tq_sh_P3_max=global
  wires:
  Power Calculation/1(P_max_EM_P3_kW) -> P_max_EM_P3_kW/1
  "Power Calculation "/1(P_kW) -> P_min_EM_P3_kW/1
  Saturation/1 -> Min/2
  1-D Lookup Table1/1 -> [tq_sh_P3_max], Gain/1, Min/1  "tq_sh_P3_lim"
  n_Upmin IN/1 -> 1-D Lookup Table1/1, Battery and Operating Strategy Limitation (Recuperation)/1(n_Upmin IN), Battery and Operating Strategy Limitation (Drive)/1(n_Upmin IN)  "n_Upmin"
  tq_sh_P3_des/1 -> Saturation/1
  Battery and Operating Strategy Limitation (Drive)/2(tq_sh_P3_bat_limted) -> P3_M_Nm_Drive/1, Power Calculation/2(tq_sh_P3_bat_limted)
  Min/1 -> Battery and Operating Strategy Limitation (Drive)/2(tq_sh_P3_limted)  "tq_sh_P3_limted"
  P_max_EM_kW/1 -> Battery and Operating Strategy Limitation (Drive)/3(P_max_EM_kW)
  Battery and Operating Strategy Limitation (Drive)/1(n_Upmin OUT) -> Power Calculation/1(n_Upmin)
  Battery and Operating Strategy Limitation (Recuperation)/2(tq_sh_P3_bat_limted) -> "Power Calculation "/2(tq_sh_P3_bat_limted), P3_M_Nm_Recu/1
  Gain/1 -> Battery and Operating Strategy Limitation (Recuperation)/2(Torque_Recu_In)
  P_min_EM_kW/1 -> Battery and Operating Strategy Limitation (Recuperation)/3(P_mech_max_kW)
  Battery and Operating Strategy Limitation (Recuperation)/1(n_Upmin OUT) -> "Power Calculation "/1(n_Upmin)

== system Simulation_Fahrmodell_v3_straight_line/Vehicle Dynamics Model /Drivetrain/Primary and Secondary Axle Powertrain Selector/Primary Axle Powertrain Selector/Hybrid Drive/P3/P3 Motor disabled ==
  n_Upmin IN : Inport
  tq_sh_P3_des : Inport  Port=2
  P_max_EM_kW : Inport  Port=3
  P_min_EM_kW : Inport  Port=4
  Constant : Constant  Value=0
  Terminator{,1..3} (4 alike) : Terminator
  P3_M_Nm_Drive : Outport
  P_max_EM_P3_kW : Outport  Port=2
  P_min_EM_P3_kW : Outport  Port=3
  P3_M_Nm_Recu : Outport  Port=4
  wires:
  Constant/1 -> P_min_EM_P3_kW/1, P_max_EM_P3_kW/1, P3_M_Nm_Drive/1, P3_M_Nm_Recu/1
  n_Upmin IN/1 -> Terminator/1  "Motordrehzahl (1/min)"
  P_max_EM_kW/1 -> Terminator1/1
  P_min_EM_kW/1 -> Terminator2/1
  tq_sh_P3_des/1 -> Terminator3/1

== system Simulation_Fahrmodell_v3_straight_line/Vehicle Dynamics Model /Drivetrain/Primary and Secondary Axle Powertrain Selector/Secondary Axle Powertrain Selector/Auswahl P4, P4_Dual-Motor/P4 // E2 Single Motor/Battery and Operating Strategy Limitation (Drive) ==
  Motordrehzahl (1/min) : Inport
  Torque_Drive_In : Inport  Port=2
  P_max_EV_kW : Inport  Port=3
  "Begrenzung BAT + Betriebsstrategie EM P4, Fahren1" : Subsystem
  Discharge Limit : Subsystem
  n_Upmin OUT : Outport
  tq_sh_P4_bat_limted : Outport  Port=2
  wires:
  Discharge Limit/1(Torque_Drive_Out) -> "Begrenzung BAT + Betriebsstrategie EM P4, Fahren1"/2(M_Nm)  "P4_M_Nm_Fahren"
  "Begrenzung BAT + Betriebsstrategie EM P4, Fahren1"/2(M_begr_Nm) -> tq_sh_P4_bat_limted/1  "P4_M_Nm_Fahren"
  P_max_EV_kW/1 -> "Begrenzung BAT + Betriebsstrategie EM P4, Fahren1"/3(P_mech_max_kW)
  Torque_Drive_In/1 -> Discharge Limit/1(Torque_Drive_In)
  Motordrehzahl (1/min)/1 -> "Begrenzung BAT + Betriebsstrategie EM P4, Fahren1"/1(n_Upmin IN)
  "Begrenzung BAT + Betriebsstrategie EM P4, Fahren1"/1(n_Upmin OUT) -> n_Upmin OUT/1

== system Simulation_Fahrmodell_v3_straight_line/Vehicle Dynamics Model /Drivetrain/Primary and Secondary Axle Powertrain Selector/Secondary Axle Powertrain Selector/Auswahl P4, P4_Dual-Motor/P4 // E2 Single Motor/Battery and Operating Strategy Limitation (Recuperation) ==
  Motordrehzahl (1/min) : Inport
  Torque_Recu_In : Inport  Port=2
  P_min_EV_kW : Inport  Port=3
  "Begrenzung BAT + Betriebsstrategie EM P4, Reku1" : Subsystem
  Recuperation Limit : Subsystem
  n_Upmin OUT : Outport
  tq_sh_P4_bat_limted_recu : Outport  Port=2
  wires:
  Recuperation Limit/1(Torque_Recu_Out) -> "Begrenzung BAT + Betriebsstrategie EM P4, Reku1"/2(M_Nm)  "P4_M_Nm_Reku"
  P_min_EV_kW/1 -> "Begrenzung BAT + Betriebsstrategie EM P4, Reku1"/3(P_mech_max_kW)
  Motordrehzahl (1/min)/1 -> "Begrenzung BAT + Betriebsstrategie EM P4, Reku1"/1(n_Upmin IN)
  "Begrenzung BAT + Betriebsstrategie EM P4, Reku1"/1(n_Upmin OUT) -> n_Upmin OUT/1
  Torque_Recu_In/1 -> Recuperation Limit/1(Torque_Recu_In)
  "Begrenzung BAT + Betriebsstrategie EM P4, Reku1"/2(M_begr_Nm) -> tq_sh_P4_bat_limted_recu/1  "P4_M_Nm_Reku"

== system Simulation_Fahrmodell_v3_straight_line/Vehicle Dynamics Model /Drivetrain/Primary and Secondary Axle Powertrain Selector/Secondary Axle Powertrain Selector/Auswahl P4, P4_Dual-Motor/P4 // E2 Single Motor/Power Calculation ==
  n_Upmin : Inport
  tq_sh_P4_bat_limted : Inport  Port=2
  Constant1 : Constant  Value=2*pi/60/1000
  Product : Product  Inputs=3
  P_kW : Outport
  wires:
  Product/1 -> P_kW/1
  n_Upmin/1 -> Product/2
  Constant1/1 -> Product/3
  tq_sh_P4_bat_limted/1 -> Product/1

== system Simulation_Fahrmodell_v3_straight_line/Vehicle Dynamics Model /Drivetrain/Primary and Secondary Axle Powertrain Selector/Secondary Axle Powertrain Selector/Auswahl P4, P4_Dual-Motor/P4 // E2 Single Motor/Power Calculation  ==
  n_Upmin : Inport
  tq_sh_P4_bat_limted_recu : Inport  Port=2
  Constant1 : Constant  Value=2*pi/60/1000
  Product : Product  Inputs=3
  P_kW : Outport
  wires:
  Product/1 -> P_kW/1
  n_Upmin/1 -> Product/2
  Constant1/1 -> Product/3
  tq_sh_P4_bat_limted_recu/1 -> Product/1

== system Simulation_Fahrmodell_v3_straight_line/Vehicle Dynamics Model /Drivetrain/Primary and Secondary Axle Powertrain Selector/Secondary Axle Powertrain Selector/Auswahl P4, P4_Dual-Motor/P4 // E3 // E4 Dual Motor/Battery and Operating Strategy Limitation (Drive) 1 ==
  Motordrehzahl (1/min) : Inport
  tq_sh_P4_DM1_limted : Inport  Port=2
  P_max_EM_kW : Inport  Port=3
  "Begrenzung BAT + Betriebsstrategie EM P4_DM_L, Fahren1" : Subsystem
  Discharge Limit1 : Subsystem
  n_Upmin OUT : Outport
  tq_sh_P4DM1_bat_limted : Outport  Port=2
  wires:
  "Begrenzung BAT + Betriebsstrategie EM P4_DM_L, Fahren1"/1(n_Upmin OUT) -> n_Upmin OUT/1
  Discharge Limit1/1(Torque_Drive_Out) -> "Begrenzung BAT + Betriebsstrategie EM P4_DM_L, Fahren1"/2(M_Nm)  "P4_M_Nm_Fahren"
  Motordrehzahl (1/min)/1 -> "Begrenzung BAT + Betriebsstrategie EM P4_DM_L, Fahren1"/1(n_Upmin IN)
  "Begrenzung BAT + Betriebsstrategie EM P4_DM_L, Fahren1"/2(M_begr_Nm) -> tq_sh_P4DM1_bat_limted/1  "P4_DM1_M_Nm_Fahren"
  P_max_EM_kW/1 -> "Begrenzung BAT + Betriebsstrategie EM P4_DM_L, Fahren1"/3(P_mech_max_kW)
  tq_sh_P4_DM1_limted/1 -> Discharge Limit1/1(Torque_Drive_In)

== system Simulation_Fahrmodell_v3_straight_line/Vehicle Dynamics Model /Drivetrain/Primary and Secondary Axle Powertrain Selector/Secondary Axle Powertrain Selector/Auswahl P4, P4_Dual-Motor/P4 // E3 // E4 Dual Motor/Battery and Operating Strategy Limitation (Drive) 2 ==
  Motordrehzahl (1/min) : Inport
  tq_sh_P4_DM2_limted : Inport  Port=2
  P_max_EM_kW : Inport  Port=3
  "Begrenzung BAT + Betriebsstrategie EM P4_DM_R, Fahren2" : Subsystem
  Discharge Limit : Subsystem
  n_Upmin OUT : Outport
  tq_sh_P4DM2_bat_limted : Outport  Port=2
  wires:
  Discharge Limit/1(Torque_Drive_Out) -> "Begrenzung BAT + Betriebsstrategie EM P4_DM_R, Fahren2"/2(M_Nm)  "P4_M_Nm_Fahren"
  "Begrenzung BAT + Betriebsstrategie EM P4_DM_R, Fahren2"/2(M_begr_Nm) -> tq_sh_P4DM2_bat_limted/1  "P4_DM2_M_Nm_Fahren"
  tq_sh_P4_DM2_limted/1 -> Discharge Limit/1(Torque_Drive_In)
  P_max_EM_kW/1 -> "Begrenzung BAT + Betriebsstrategie EM P4_DM_R, Fahren2"/3(P_mech_max_kW)
  Motordrehzahl (1/min)/1 -> "Begrenzung BAT + Betriebsstrategie EM P4_DM_R, Fahren2"/1(n_Upmin IN)
  "Begrenzung BAT + Betriebsstrategie EM P4_DM_R, Fahren2"/1(n_Upmin OUT) -> n_Upmin OUT/1

== system Simulation_Fahrmodell_v3_straight_line/Vehicle Dynamics Model /Drivetrain/Primary and Secondary Axle Powertrain Selector/Secondary Axle Powertrain Selector/Auswahl P4, P4_Dual-Motor/P4 // E3 // E4 Dual Motor/Battery and Operating Strategy Limitation (Recuperation) 1 ==
  Motordrehzahl (1/min) : Inport
  Torque_Recu_In : Inport  Port=2
  P_min_EM_kW : Inport  Port=3
  "Begrenzung BAT + Betriebsstrategie EM P4_DM_L, Reku1" : Subsystem
  Recuperation Limit1 : Subsystem
  n_Upmin OUT : Outport
  tq_sh_P4DM1_bat_limted_recu : Outport  Port=2
  wires:
  Recuperation Limit1/1(Torque_Recu_Out) -> "Begrenzung BAT + Betriebsstrategie EM P4_DM_L, Reku1"/2(M_Nm)  "P4_M_Nm_Reku"
  "Begrenzung BAT + Betriebsstrategie EM P4_DM_L, Reku1"/1(n_Upmin OUT) -> n_Upmin OUT/1
  P_min_EM_kW/1 -> "Begrenzung BAT + Betriebsstrategie EM P4_DM_L, Reku1"/3(P_mech_max_kW)
  Motordrehzahl (1/min)/1 -> "Begrenzung BAT + Betriebsstrategie EM P4_DM_L, Reku1"/1(n_Upmin IN)
  "Begrenzung BAT + Betriebsstrategie EM P4_DM_L, Reku1"/2(M_begr_Nm) -> tq_sh_P4DM1_bat_limted_recu/1  "P4_DM1_M_Nm_Reku"
  Torque_Recu_In/1 -> Recuperation Limit1/1(Torque_Recu_In)

== system Simulation_Fahrmodell_v3_straight_line/Vehicle Dynamics Model /Drivetrain/Primary and Secondary Axle Powertrain Selector/Secondary Axle Powertrain Selector/Auswahl P4, P4_Dual-Motor/P4 // E3 // E4 Dual Motor/Battery and Operating Strategy Limitation (Recuperation) 2 ==
  Motordrehzahl (1/min) : Inport
  Torque_Recu_In : Inport  Port=2
  P_min_EM_kW : Inport  Port=3
  "Begrenzung BAT + Betriebsstrategie EM P4_DM_R, Reku2" : Subsystem
  Recuperation Limit : Subsystem
  n_Upmin OUT : Outport
  tq_sh_P4DM2_bat_limted_recu : Outport  Port=2
  wires:
  Recuperation Limit/1(Torque_Recu_Out) -> "Begrenzung BAT + Betriebsstrategie EM P4_DM_R, Reku2"/2(M_Nm)  "P4_M_Nm_Reku"
  Motordrehzahl (1/min)/1 -> "Begrenzung BAT + Betriebsstrategie EM P4_DM_R, Reku2"/1(n_Upmin IN)
  P_min_EM_kW/1 -> "Begrenzung BAT + Betriebsstrategie EM P4_DM_R, Reku2"/3(P_mech_max_kW)
  Torque_Recu_In/1 -> Recuperation Limit/1(Torque_Recu_In)
  "Begrenzung BAT + Betriebsstrategie EM P4_DM_R, Reku2"/1(n_Upmin OUT) -> n_Upmin OUT/1
  "Begrenzung BAT + Betriebsstrategie EM P4_DM_R, Reku2"/2(M_begr_Nm) -> tq_sh_P4DM2_bat_limted_recu/1  "P4_DM2_M_Nm_Reku"

== system Simulation_Fahrmodell_v3_straight_line/Vehicle Dynamics Model /Drivetrain/Primary and Secondary Axle Powertrain Selector/Secondary Axle Powertrain Selector/Auswahl P4, P4_Dual-Motor/P4 // E3 // E4 Dual Motor/Power Calculation  ==
  n_Upmin : Inport
  tq_sh_P4DM2_bat_limted_recu : Inport  Port=2
  Constant1 : Constant  Value=2*pi/60/1000
  Product : Product  Inputs=3
  P_kW : Outport
  wires:
  Product/1 -> P_kW/1
  n_Upmin/1 -> Product/2
  Constant1/1 -> Product/3
  tq_sh_P4DM2_bat_limted_recu/1 -> Product/1

== system Simulation_Fahrmodell_v3_straight_line/Vehicle Dynamics Model /Drivetrain/Primary and Secondary Axle Powertrain Selector/Secondary Axle Powertrain Selector/Auswahl P4, P4_Dual-Motor/P4 // E3 // E4 Dual Motor/Power Calculation    ==
  n_Upmin : Inport
  tq_sh_P4DM2_bat_limted : Inport  Port=2
  Constant1 : Constant  Value=2*pi/60/1000
  Product : Product  Inputs=3
  P_kW : Outport
  wires:
  Product/1 -> P_kW/1
  n_Upmin/1 -> Product/2
  Constant1/1 -> Product/3
  tq_sh_P4DM2_bat_limted/1 -> Product/1

== system Simulation_Fahrmodell_v3_straight_line/Vehicle Dynamics Model /Drivetrain/Primary and Secondary Axle Powertrain Selector/Secondary Axle Powertrain Selector/Auswahl P4, P4_Dual-Motor/P4 // E3 // E4 Dual Motor/Power Calculation     ==
  n_Upmin : Inport
  tq_sh_P4DM1_bat_limted_recu : Inport  Port=2
  Constant1 : Constant  Value=2*pi/60/1000
  Product : Product  Inputs=3
  P_kW : Outport
  wires:
  Product/1 -> P_kW/1
  n_Upmin/1 -> Product/2
  Constant1/1 -> Product/3
  tq_sh_P4DM1_bat_limted_recu/1 -> Product/1

== system Simulation_Fahrmodell_v3_straight_line/Vehicle Dynamics Model /Drivetrain/Primary and Secondary Axle Powertrain Selector/Secondary Axle Powertrain Selector/Auswahl P4, P4_Dual-Motor/P4 // E3 // E4 Dual Motor/Power Calculation      ==
  n_Upmin : Inport
  tq_sh_P4DM1_bat_limted : Inport  Port=2
  Constant1 : Constant  Value=2*pi/60/1000
  Product : Product  Inputs=3
  P_kW : Outport
  wires:
  Product/1 -> P_kW/1
  n_Upmin/1 -> Product/2
  Constant1/1 -> Product/3
  tq_sh_P4DM1_bat_limted/1 -> Product/1

== system Simulation_Fahrmodell_v3_straight_line/Vehicle Dynamics Model /Drivetrain/Primary and Secondary Axle Powertrain Selector/Primary Axle Powertrain Selector/Electric Drive/Variant Subsystem/EV Dual Motor/Battery and Operating Strategy Limitation (Drive) ==
  Motordrehzahl (1/min) : Inport
  tq_sh_EV_DM1_limted : Inport  Port=2
  "Begrenzung BAT + Betriebsstrategie EM P4_DM_L, Fahren2" : Subsystem
  Discharge Limit : Subsystem
  n_Upmin OUT : Outport
  tq_sh_EV_DM1_bat_limted : Outport  Port=2
  wires:
  Motordrehzahl (1/min)/1 -> "Begrenzung BAT + Betriebsstrategie EM P4_DM_L, Fahren2"/1(n_Upmin IN)
  Discharge Limit/1(Torque_Drive_Out) -> "Begrenzung BAT + Betriebsstrategie EM P4_DM_L, Fahren2"/2(M_Nm)  "P4_M_Nm_Fahren"
  [P_max_EM_kW] -> "Begrenzung BAT + Betriebsstrategie EM P4_DM_L, Fahren2"/3(P_mech_max_kW)  "P_max_EM_kW"
  "Begrenzung BAT + Betriebsstrategie EM P4_DM_L, Fahren2"/2(M_begr_Nm) -> tq_sh_EV_DM1_bat_limted/1  "EV_DM1_M_Nm_Fahren"
  "Begrenzung BAT + Betriebsstrategie EM P4_DM_L, Fahren2"/1(n_Upmin OUT) -> n_Upmin OUT/1
  tq_sh_EV_DM1_limted/1 -> Discharge Limit/1(Torque_Drive_In)

== system Simulation_Fahrmodell_v3_straight_line/Vehicle Dynamics Model /Drivetrain/Primary and Secondary Axle Powertrain Selector/Primary Axle Powertrain Selector/Electric Drive/Variant Subsystem/EV Dual Motor/Battery and Operating Strategy Limitation (Drive)  ==
  Motordrehzahl (1/min) : Inport
  tq_sh_EV_DM2_limted : Inport  Port=2
  "Begrenzung BAT + Betriebsstrategie EM P4_DM_R, Fahren1" : Subsystem
  Discharge Limit1 : Subsystem
  n_Upmin OUT : Outport
  tq_sh_EV_DM2_bat_limted : Outport  Port=2
  wires:
  [P_max_EM_kW] -> "Begrenzung BAT + Betriebsstrategie EM P4_DM_R, Fahren1"/3(P_mech_max_kW)  "P_max_EM_kW"
  "Begrenzung BAT + Betriebsstrategie EM P4_DM_R, Fahren1"/1(n_Upmin OUT) -> n_Upmin OUT/1
  Motordrehzahl (1/min)/1 -> "Begrenzung BAT + Betriebsstrategie EM P4_DM_R, Fahren1"/1(n_Upmin IN)
  Discharge Limit1/1(Torque_Drive_Out) -> "Begrenzung BAT + Betriebsstrategie EM P4_DM_R, Fahren1"/2(M_Nm)  "P4_M_Nm_Fahren"
  tq_sh_EV_DM2_limted/1 -> Discharge Limit1/1(Torque_Drive_In)
  "Begrenzung BAT + Betriebsstrategie EM P4_DM_R, Fahren1"/2(M_begr_Nm) -> tq_sh_EV_DM2_bat_limted/1  "P4_DM2_M_Nm_Fahren"

== system Simulation_Fahrmodell_v3_straight_line/Vehicle Dynamics Model /Drivetrain/Primary and Secondary Axle Powertrain Selector/Primary Axle Powertrain Selector/Electric Drive/Variant Subsystem/EV Dual Motor/Battery and Operating Strategy Limitation (Recuperation) ==
  Motordrehzahl (1/min) : Inport
  Torque_Recu_In : Inport  Port=2
  "Begrenzung BAT + Betriebsstrategie EM P4_DM_L, Reku2" : Subsystem
  Recuperation Limit1 : Subsystem
  n_Upmin OUT : Outport
  tq_sh_EV_DM1_bat_limted_recu : Outport  Port=2
  wires:
  "Begrenzung BAT + Betriebsstrategie EM P4_DM_L, Reku2"/2(M_begr_Nm) -> tq_sh_EV_DM1_bat_limted_recu/1  "EV_DM1_M_Nm_Reku"
  [P_min_EM_kW] -> "Begrenzung BAT + Betriebsstrategie EM P4_DM_L, Reku2"/3(P_mech_max_kW)  "P_min_EM_kW"
  Recuperation Limit1/1(Torque_Recu_Out) -> "Begrenzung BAT + Betriebsstrategie EM P4_DM_L, Reku2"/2(M_Nm)  "P4_M_Nm_Reku"
  Motordrehzahl (1/min)/1 -> "Begrenzung BAT + Betriebsstrategie EM P4_DM_L, Reku2"/1(n_Upmin IN)
  "Begrenzung BAT + Betriebsstrategie EM P4_DM_L, Reku2"/1(n_Upmin OUT) -> n_Upmin OUT/1
  Torque_Recu_In/1 -> Recuperation Limit1/1(Torque_Recu_In)

== system Simulation_Fahrmodell_v3_straight_line/Vehicle Dynamics Model /Drivetrain/Primary and Secondary Axle Powertrain Selector/Primary Axle Powertrain Selector/Electric Drive/Variant Subsystem/EV Dual Motor/Battery and Operating Strategy Limitation (Recuperation)  ==
  Motordrehzahl (1/min) : Inport
  Torque_Recu_In : Inport  Port=2
  "Begrenzung BAT + Betriebsstrategie EM P4_DM_R, Reku1" : Subsystem
  Recuperation Limit : Subsystem
  n_Upmin OUT : Outport
  tq_sh_EV_DM2_bat_limted_recu : Outport  Port=2
  wires:
  "Begrenzung BAT + Betriebsstrategie EM P4_DM_R, Reku1"/2(M_begr_Nm) -> tq_sh_EV_DM2_bat_limted_recu/1  "EV_DM2_M_Nm_Reku"
  [P_min_EM_kW] -> "Begrenzung BAT + Betriebsstrategie EM P4_DM_R, Reku1"/3(P_mech_max_kW)  "P_min_EM_kW"
  "Begrenzung BAT + Betriebsstrategie EM P4_DM_R, Reku1"/1(n_Upmin OUT) -> n_Upmin OUT/1
  Recuperation Limit/1(Torque_Recu_Out) -> "Begrenzung BAT + Betriebsstrategie EM P4_DM_R, Reku1"/2(M_Nm)  "P4_M_Nm_Reku"
  Torque_Recu_In/1 -> Recuperation Limit/1(Torque_Recu_In)
  Motordrehzahl (1/min)/1 -> "Begrenzung BAT + Betriebsstrategie EM P4_DM_R, Reku1"/1(n_Upmin IN)

== system Simulation_Fahrmodell_v3_straight_line/Vehicle Dynamics Model /Drivetrain/Primary and Secondary Axle Powertrain Selector/Primary Axle Powertrain Selector/Electric Drive/Variant Subsystem/EV Dual Motor/Power Calculation ==
  n_Upmin : Inport
  tq_sh_EV_DM2_bat_limted_recu : Inport  Port=2
  Constant1 : Constant  Value=2*pi/60/1000
  Product : Product  Inputs=3
  P_kW : Outport
  wires:
  Product/1 -> P_kW/1
  n_Upmin/1 -> Product/2
  Constant1/1 -> Product/3
  tq_sh_EV_DM2_bat_limted_recu/1 -> Product/1

== system Simulation_Fahrmodell_v3_straight_line/Vehicle Dynamics Model /Drivetrain/Primary and Secondary Axle Powertrain Selector/Primary Axle Powertrain Selector/Electric Drive/Variant Subsystem/EV Dual Motor/Power Calculation  ==
  n_Upmin : Inport
  tq_sh_EV_DM1_bat_limted : Inport  Port=2
  Constant1 : Constant  Value=2*pi/60/1000
  Product : Product  Inputs=3
  P_kW : Outport
  wires:
  Product/1 -> P_kW/1
  n_Upmin/1 -> Product/2
  Constant1/1 -> Product/3
  tq_sh_EV_DM1_bat_limted/1 -> Product/1
